simulink model "measures"  (R2016a)
settings: Solver=FixedStepAuto  SolverMode=SingleTasking  StartTime=0.0  StopTime=3  FixedStep=0.01  RelTol=1e-3
settings Model: Creator=Shayan  LastModifiedBy=Shayan
settings DebuggingCC: SFUnexpectedBacktrackingDiag=error  SFNoUnconditionalDefaultTransitionDiag=error
settings SFSimCC: SimUseLocalCustomCode=on
settings RTWCC: RTWUseLocalCustomCode=on
settings GRTTargetCC: TargetLangStandard=C99 (ISO)  GeneratePreprocessorConditionals=Use local settings
settings ConfigComp: CovMetricSettings=dwe  CovHtmlReporting=off  CovSaveCumulativeToWorkspaceVar=off  CovSaveSingleToWorkspaceVar=off  CovExternalEMLEnable=on

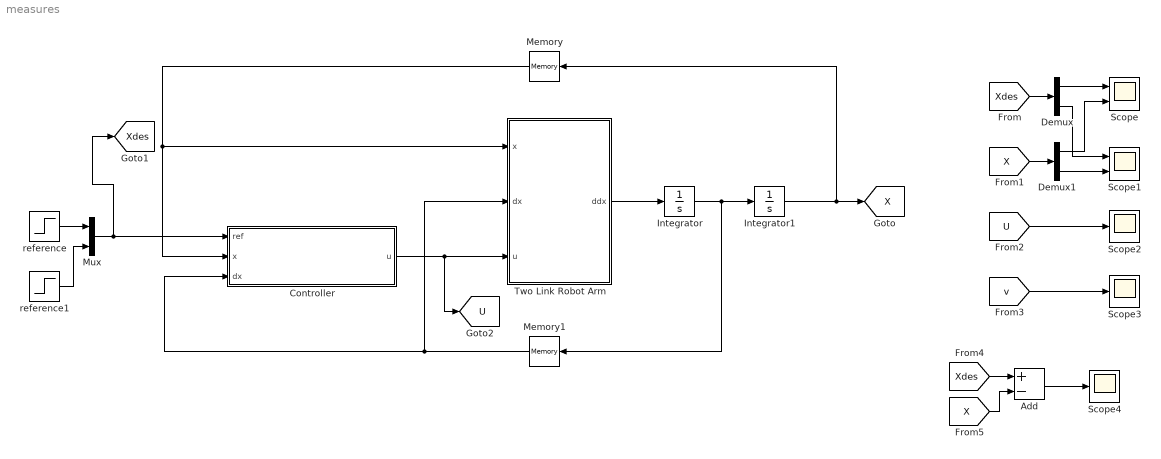
== system measures ==
  Add : Sum  Inputs=+-
  Controller : Subsystem
  Demux : Demux  Outputs=2
  Demux1 : Demux  Outputs=2
  Integrator : Integrator  InitialCondition=[0 0]
  Integrator1 : Integrator  InitialCondition=[pi/2 -pi/2]
  Memory : Memory  X0=[pi/2 -pi/2]
  Memory1 : Memory  X0=[0 0]
  Mux : Mux  Inputs=2
  Scope : Scope  NumInputPorts=2
  Scope1 : Scope  NumInputPorts=2
  Scope2 : Scope
  Scope3 : Scope
  Scope4 : Scope
  Two Link Robot Arm : MATLAB Function  TreatAsAtomicUnit=on
  reference : Step  Time=0  After=-pi/2  SampleTime=0
  reference1 : Step  Time=0  After=pi/2  SampleTime=0
  tag scope: U=global, X=global, Xdes=global
  wires:
  Integrator/1 -> Memory1/1, Integrator1/1
  Two Link Robot Arm/1(ddx) -> Integrator/1
  Integrator1/1 -> [X], Memory/1
  Memory/1 -> Two Link Robot Arm/1(x), Controller/2(x)
  Memory1/1 -> Controller/3(dx), Two Link Robot Arm/2(dx)
  reference/1 -> Mux/1
  reference1/1 -> Mux/2
  Mux/1 -> [Xdes], Controller/1(ref)
  Controller/1(u) -> [U], Two Link Robot Arm/3(u)
  [Xdes] -> Demux/1
  [X] -> Demux1/1
  Demux/1 -> Scope/1
  Demux1/1 -> Scope/2
  Demux1/2 -> Scope1/2
  Demux/2 -> Scope1/1
  [U] -> Scope2/1
  [v] -> Scope3/1
  [Xdes] -> Add/1
  [X] -> Add/2
  Add/1 -> Scope4/1

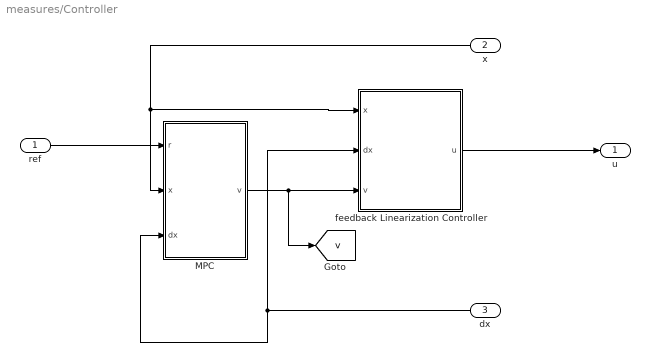
== system measures/Controller ==
  ref : Inport
  x : Inport  Port=2
  dx : Inport  Port=3
  MPC : MATLAB Function  TreatAsAtomicUnit=on
  feedback Linearization Controller : MATLAB Function  TreatAsAtomicUnit=on
  u : Outport
  tag scope: v=global
  wires:
  ref/1 -> MPC/1(r)
  x/1 -> feedback Linearization Controller/1(x), MPC/2(x)
  MPC/1(v) -> [v], feedback Linearization Controller/3(v)
  dx/1 -> feedback Linearization Controller/2(dx), MPC/3(dx)
  feedback Linearization Controller/1(u) -> u/1

== matlab function measures/Controller/feedback Linearization Controller ==
  data: x input; dx input; u output; v input
function u = fcn(x,dx,v)

M1 = 1;
M2 = 1;
L1 = 1;
L2 = 1;
g = 9.81;
G = [-(M1+M2)*g*L1-M2*g*L2*sin(x(1)+x(2));...
    -M2*g*L2*sin(x(1)+x(2));];
C = [M1*L1*L2*(2*dx(1)*dx(2) + dx(1)^2)*sin(x(2));...
    -M2*L1*L2*dx(1)*dx(2)*sin(x(2));];
M = [-(M1+M2)*L1^2 + M2*L2^2 + 2*M2*L1*L2*cos(x(2)), M2*L2^2 + M2*L1*L2*cos(x(2));...
     M2*L2^2 + M2*L1*L2*cos(x(2)),  M2*L2^2;];



u = M*v + C + G;

== matlab function measures/Two Link Robot Arm ==
  data: x input; dx input; u input; ddx output
function ddx = fcn(x,dx,u)

M1 = 1;
M2 = 1;
L1 = 1;
L2 = 1;
g = 9.81;
G = [-(M1+M2)*g*L1-M2*g*L2*sin(x(1)+x(2));...
    -M2*g*L2*sin(x(1)+x(2));];
C = [M1*L1*L2*(2*dx(1)*dx(2) + dx(1)^2)*sin(x(2));...
    -M2*L1*L2*dx(1)*dx(2)*sin(x(2));];
M = [-(M1+M2)*L1^2 + M2*L2^2 + 2*M2*L1*L2*cos(x(2)), M2*L2^2 + M2*L1*L2*cos(x(2));...
     M2*L2^2 + M2*L1*L2*cos(x(2)),  M2*L2^2;];
ddx = inv(M)*(-C-G+u);

== matlab function measures/Controller/MPC ==
  data: r input; v output; x input; dx input
function v  = fcn(r,x,dx)

k1 = 15.99;
k2 = 5.65;
k3 = k1;

v = [k3*r(1) - k1*x(1) - k2*dx(1);...
     (k3*r(2) - k1*x(2) - k2*dx(2));];
